simulink model "adcs_actuator"  (R2024b)
settings: Solver=VariableStepAuto  StartTime=0.0  StopTime=10.0  RelTol=1e-3
settings Model: DataDictionary=adcs_params.sldd  Creator=natha  LastModifiedBy=natha

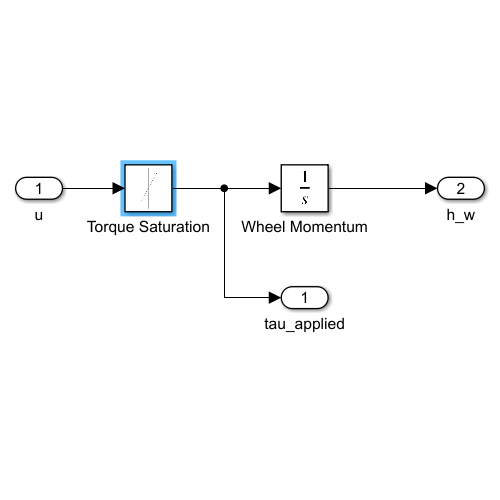
[thumbnail: Simulink's stored preview of the top-level diagram]
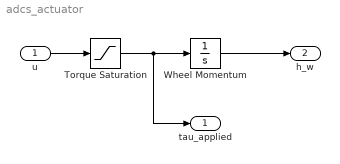
== system adcs_actuator ==
  u : Inport  PortDimensions=3
  Torque Saturation : Saturate  UpperLimit=100  LowerLimit=-100
  Wheel Momentum : Integrator  InitialCondition=[0;0;0]
  tau_applied : Outport  PortDimensions=3
  h_w : Outport  Port=2  PortDimensions=3
  wires:
  u/1 -> Torque Saturation/1
  Torque Saturation/1 -> tau_applied/1, Wheel Momentum/1
  Wheel Momentum/1 -> h_w/1
